simulink model "qfdfir_poc"  (Simulink 7.0)
settings: Solver=ode45  StartTime=0.0  StopTime=1e4  RelTol=1e-3
libraries: xbsIndex_r4 x15, simulink x1
settings Model: Creator=mdexter  LastModifiedBy=mdexter

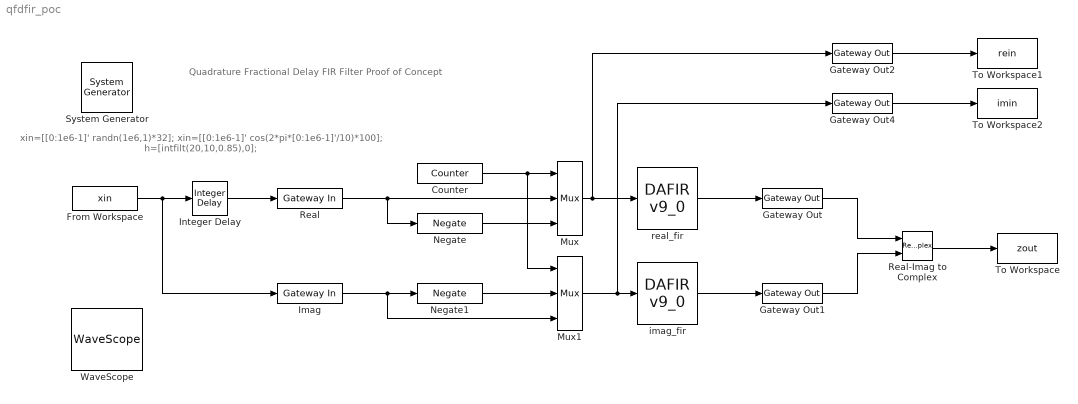
== system qfdfir_poc ==
  note: Quadrature Fractional Delay FIR Filter
      | Proof of Concept
  note: xin=[[0:1e6-1]' randn(1e6,1)*32];
      | xin=[[0:1e6-1]' cos(2*pi*[0:1e6-1]'/10)*100];
      | h=[intfilt(20,10,0.85),0];
  " System Generator" : xbsIndex_r4/ System Generator  Tag=genX  SystemSampleTime=-1  xilinxfamily=Virtex4  part=xc4vsx35  speed=-10  package=ff668  synthesis_tool=XST  clock_wrapper=Clock Enables  directory=./netlist  testbench=off  simulink_period=1  sysclk_period=100  dcm_input_clock_period=100  incr_netlist=off  trim_vbits=Everywhere in SubSystem  dbl_ovrd=According to Block Masks  core_generation=According to Block Masks  run_coregen=off  deprecated_control=off  eval_field=0  block_type=sysgen
      settings: block_version=10.1.3
  Counter : xbsIndex_r4/Counter  cnt_type=Free Running  cnt_to=Inf  operation=Up  start_count=1  cnt_by_val=1  arith_type=Unsigned  n_bits=1  bin_pt=0  load_pin=off  rst=off  en=off  explicit_period=on  period=2  dbl_ovrd=off  use_behavioral_HDL=off  use_rpm=off  implementation=Fabric  block_type=counter
  From Workspace : FromWorkspace  VariableName=xin  SampleTime=1  Interpolate=off  OutputAfterFinalValue=Holding final value
  Gateway Out{,1..2,4} (4 alike) : xbsIndex_r4/Gateway Out  hdl_port=on  timing_constraint=None  locs_specified=off  LOCs={}  block_type=gatewayout
      settings: infoedit="Gateway out block.  Converts Xilinx fixed point inputs into ouputs of type Simulink integer, double, or fixed point.<P><P>Hardware notes:  In hardware these blocks become top level output ports or are discarded, depending on how they are configured."  block_version=10.1.3
  Imag : xbsIndex_r4/Gateway In  arith_type="Signed  (2's comp)"  n_bits=8  bin_pt=0  quantization="Round  (unbiased: +/- Inf)"  overflow=Saturate  period=2  dbl_ovrd=off  timing_constraint=None  locs_specified=off  LOCs={}  block_type=gatewayin
      settings: infoedit="Gateway in block.  Converts inputs of type Simulink integer, double and fixed point to  Xilinx fixed point type.<P><P>Hardware notes:  In hardware these blocks become top level input ports."  block_version=10.1.3
  Integer Delay : simulink/Discrete/Integer Delay  vinit=0.0  samptime=-1  NumDelays=1
  Mux : xbsIndex_r4/Mux  inputs=2  en=off  latency=0  precision=Full  arith_type=Unsigned  n_bits=16  bin_pt=14  quantization=Truncate  overflow=Wrap  dbl_ovrd=off  block_type=mux
  Mux1 : xbsIndex_r4/Mux  inputs=2  en=off  latency=0  precision=Full  arith_type=Unsigned  n_bits=16  bin_pt=14  quantization=Truncate  overflow=Wrap  dbl_ovrd=off  block_type=mux
  Negate : xbsIndex_r4/Negate  precision=User Defined  arith_type="Signed  (2's comp)"  n_bits=8  bin_pt=0  quantization=Truncate  overflow=Saturate  en=off  latency=0  dbl_ovrd=off  block_type=negate
      settings: block_version=10.1.3
  Negate1 : xbsIndex_r4/Negate  precision=User Defined  arith_type="Signed  (2's comp)"  n_bits=8  bin_pt=0  quantization=Truncate  overflow=Saturate  en=off  latency=0  dbl_ovrd=off  block_type=negate
      settings: block_version=10.1.3
  Real : xbsIndex_r4/Gateway In  arith_type="Signed  (2's comp)"  n_bits=8  bin_pt=0  quantization="Round  (unbiased: +/- Inf)"  overflow=Saturate  period=2  dbl_ovrd=off  timing_constraint=None  locs_specified=off  LOCs={}  block_type=gatewayin
      settings: infoedit="Gateway in block.  Converts inputs of type Simulink integer, double and fixed point to  Xilinx fixed point type.<P><P>Hardware notes:  In hardware these blocks become top level input ports."  block_version=10.1.3
  Real-Imag to Complex : RealImagToComplex
  To Workspace : ToWorkspace  VariableName=zout  SampleTime=2  SaveFormat=Array
  To Workspace1 : ToWorkspace  VariableName=rein  SampleTime=2  SaveFormat=Array
  To Workspace2 : ToWorkspace  VariableName=imin  SampleTime=2  SaveFormat=Array
  WaveScope : xbsIndex_r4/WaveScope  block_type=wavescope
      settings: block_version=10.1.3
  imag_fir : xbsIndex_r4/DAFIR v9_0   coef=h(4:20:end)  structure=None  coef_n_bits=16  coef_bin_pt=14  over_sample=1  reload=off  valids=off  rst=off  latency=1  num_channels=1  serial_input=off  polyphase_behavior="Single Rate:  sample in - sample out"  dbl_ovrd=off  explicit_period=off  period=1  use_isim=0  block_type=fir
      settings: infoedit="Hardware notes: Implemented using distributed arithmetic (DA).  The hardware over sampling rate determines the degree of parallelism.  A rate of one produces a fully parallel DA filter.  A rate of n (resp., n+1) for an n-bit input signal produces a fully serial implementation for a non-symmetric (resp., symmetric) impulse response.  Intermediate values produce implementations with intermediate levels of parallelism."  block_version=10.1.3
  real_fir : xbsIndex_r4/DAFIR v9_0   coef=h(14:20:end)  structure=None  coef_n_bits=16  coef_bin_pt=14  over_sample=1  reload=off  valids=off  rst=off  latency=1  num_channels=1  serial_input=off  polyphase_behavior="Single Rate:  sample in - sample out"  dbl_ovrd=off  explicit_period=off  period=1  use_isim=0  block_type=fir
      settings: infoedit="Hardware notes: Implemented using distributed arithmetic (DA).  The hardware over sampling rate determines the degree of parallelism.  A rate of one produces a fully parallel DA filter.  A rate of n (resp., n+1) for an n-bit input signal produces a fully serial implementation for a non-symmetric (resp., symmetric) impulse response.  Intermediate values produce implementations with intermediate levels of parallelism."  block_version=10.1.3
  wires:
  From Workspace/1 -> Integer Delay/1, Imag/1
  real_fir/1 -> Gateway Out/1
  Real/1 -> Mux/2, Negate/1
  Imag/1 -> Negate1/1, Mux1/3
  Integer Delay/1 -> Real/1
  Negate/1 -> Mux/3
  Counter/1 -> Mux/1, Mux1/1
  Mux/1 -> real_fir/1, Gateway Out2/1
  Mux1/1 -> imag_fir/1, Gateway Out4/1
  Negate1/1 -> Mux1/2
  imag_fir/1 -> Gateway Out1/1
  Real-Imag to Complex/1 -> To Workspace/1
  Gateway Out/1 -> Real-Imag to Complex/1
  Gateway Out1/1 -> Real-Imag to Complex/2
  Gateway Out4/1 -> To Workspace2/1
  Gateway Out2/1 -> To Workspace1/1
